simulink model "Microgrid"  (R2026a)
settings: Solver=ode3  StopTime=86400  FixedStep=3600
settings Model: Creator=S.THANUJ  LastModifiedBy=S.THANUJ

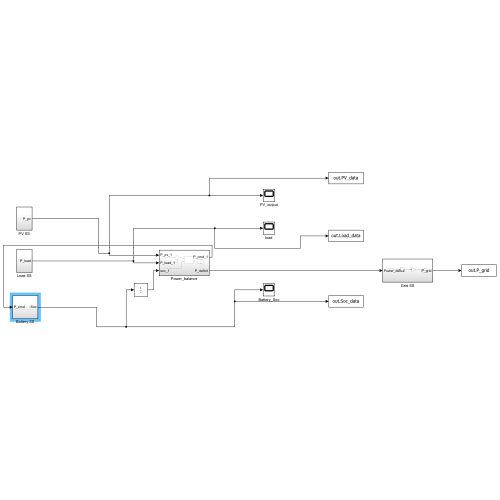
[thumbnail: Simulink's stored preview of the top-level diagram]
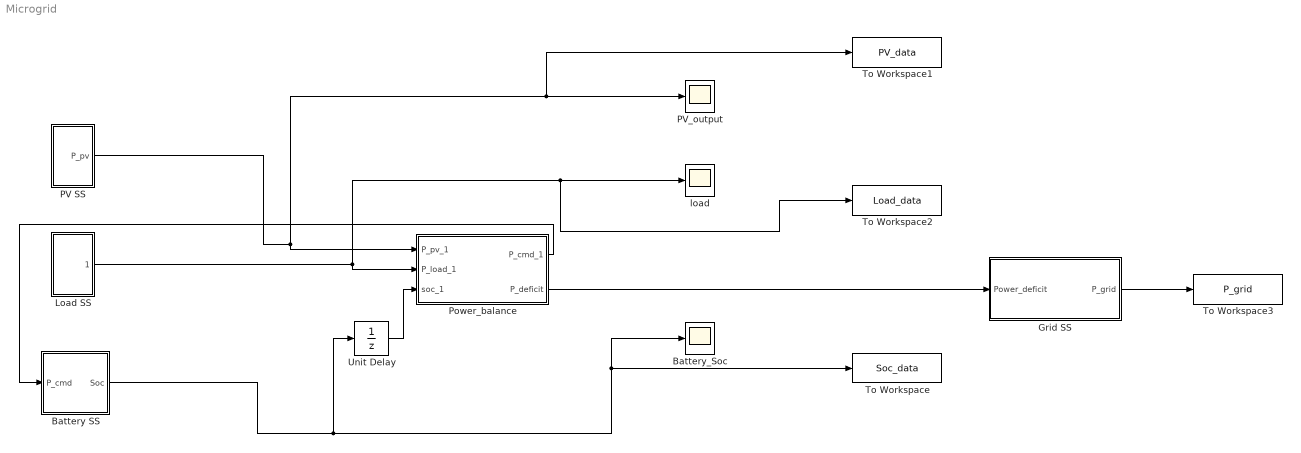
== system Microgrid ==
  Battery SS : Subsystem
  Battery_Soc : Scope
      settings: ActiveDisplayYMinimum=-1  ActiveDisplayYMaximum=1  DataLoggingVariableName=ScopeData2
  Grid SS : Subsystem
  Load SS : Subsystem
  PV SS : Subsystem
  PV_output : Scope
      settings: ActiveDisplayYMinimum=-0.001125  ActiveDisplayYMaximum=0.010125000000000002
  Power_balance : Subsystem
  To Workspace : ToWorkspace  VariableName=Soc_data  SaveFormat=Timeseries  SampleTime=-1
  To Workspace1 : ToWorkspace  VariableName=PV_data  SaveFormat=Timeseries  SampleTime=-1
  To Workspace2 : ToWorkspace  VariableName=Load_data  SaveFormat=Timeseries  SampleTime=-1
  To Workspace3 : ToWorkspace  VariableName=P_grid  SaveFormat=Timeseries  SampleTime=-1
  Unit Delay : UnitDelay  InitialCondition=0.5  SampleTime=3600
  load : Scope
      settings: ActiveDisplayYMinimum=-1  ActiveDisplayYMaximum=1
  wires:
  PV SS/1(P_pv) -> To Workspace1/1, PV_output/1, Power_balance/1(P_pv_1)
  Load SS/1(P_load) -> To Workspace2/1, load/1, Power_balance/2(P_load_1)
  Battery SS/1(Soc) -> Unit Delay/1, Battery_Soc/1, To Workspace/1
  Power_balance/1(P_cmd_1) -> Battery SS/1(P_cmd)
  Unit Delay/1 -> Power_balance/3(soc_1)
  Grid SS/1(P_grid) -> To Workspace3/1
  Power_balance/2(P_deficit) -> Grid SS/1(Power_deficit)

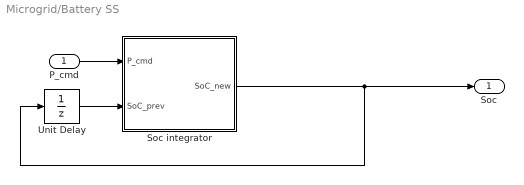
== system Microgrid/Battery SS ==
  P_cmd : Inport
  Soc integrator : MATLAB Function  TreatAsAtomicUnit=on
  Unit Delay : UnitDelay  InitialCondition=0.5  SampleTime=3600
  Soc : Outport
  wires:
  P_cmd/1 -> Soc integrator/1(P_cmd)
  Soc integrator/1(SoC_new) -> Unit Delay/1, Soc/1
  Unit Delay/1 -> Soc integrator/2(SoC_prev)

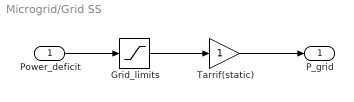
== system Microgrid/Grid SS ==
  Power_deficit : Inport
  Grid_limits : Saturate
  Tarrif(static) : Gain
  P_grid : Outport
  wires:
  Tarrif(static)/1 -> P_grid/1
  Grid_limits/1 -> Tarrif(static)/1
  Power_deficit/1 -> Grid_limits/1

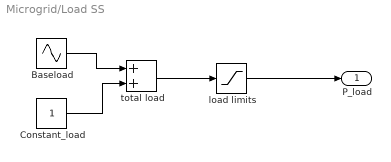
== system Microgrid/Load SS ==
  Baseload : Sin  Amplitude=6  SampleTime=0
  Constant_load : Constant
  load limits : Saturate  UpperLimit=inf  LowerLimit=0.5
  total load : Sum
  P_load : Outport
  wires:
  Baseload/1 -> total load/1
  Constant_load/1 -> total load/2
  load limits/1 -> P_load/1
  total load/1 -> load limits/1

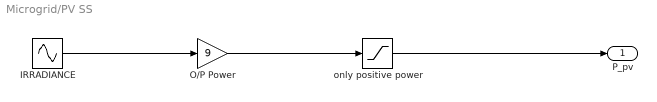
== system Microgrid/PV SS ==
  IRRADIANCE : Sin  Frequency=pi/43200  Phase=-pi/2  SampleTime=3600
  O/P Power : Gain  Gain=9
  only positive power : Saturate  UpperLimit=inf  LowerLimit=0
  P_pv : Outport
  wires:
  IRRADIANCE/1 -> O/P Power/1
  O/P Power/1 -> only positive power/1
  only positive power/1 -> P_pv/1

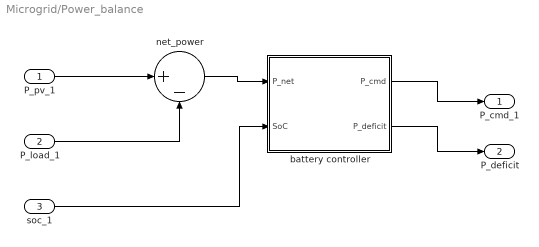
== system Microgrid/Power_balance ==
  P_pv_1 : Inport
  P_load_1 : Inport  Port=2
  soc_1 : Inport  Port=3
  battery controller : MATLAB Function  TreatAsAtomicUnit=on
  net_power : Sum  Inputs=|+-
  P_cmd_1 : Outport
  P_deficit : Outport  Port=2
  wires:
  net_power/1 -> battery controller/1(P_net)
  battery controller/1(P_cmd) -> P_cmd_1/1
  P_pv_1/1 -> net_power/1
  P_load_1/1 -> net_power/2
  soc_1/1 -> battery controller/2(SoC)
  battery controller/2(P_deficit) -> P_deficit/1

== matlab function Microgrid/Battery SS/Soc integrator ==
  data: P_cmd input; SoC_new output; SoC_prev input
function SoC_new = SoC_update(P_cmd, SoC_prev)
SoC_new = SoC_prev + P_cmd/10;
SoC_new = max(0.2, min(0.9, SoC_new));
end

== matlab function Microgrid/Power_balance/battery controller ==
  data: P_net input; P_cmd output; SoC input; P_deficit output
function [P_cmd, P_deficit] = battery_controller(P_net, SoC)
max_power = 5;

if P_net > 0 && SoC < 0.9
    P_cmd = min(P_net, max_power);
    P_deficit = 0;
elseif P_net < 0 && SoC > 0.2
    P_cmd = max(P_net, -max_power);
    P_deficit = 0;
else
    P_cmd = 0;
    P_deficit = max(0, -P_net);  % unmet load
end
end
